simulink model "Encoder_reader_simulink"  (R2025b)
settings: Solver=FixedStepAuto  StartTime=0.0  StopTime=inf  FixedStep=0.0001  RelTol=1e-3  EnableMultiTasking=on
libraries: stm32f4xxblockslib x3, stm32g4xxblockslib x3
settings Model: STM32="{\"EncoderBlockForG4\":[{\"ID\":\"untitled:1\"},{\"ID\":\"Lab3_Encoder:1\"},{\"ID\":\"Encoder_reader_simulink:1\"},{\"ID\":\"Encoder_reader_simulink:58\"},{\"ID\":\"Encoder_reader_simulink:64\"}],\"DigitalPortRead\":[{\"ID\":\"Encoder_reader_simulink:27\"},{\"ID\":\"Encoder_reader_simulink:61\"},{\"ID\":\"Encoder_reader_simulink:62\"}]}"  Creator=User  LastModifiedBy=Asus
settings OptimizationCC: DefaultParameterBehavior=Inlined  EnhancedBackFolding=on  PassReuseOutputArgsAs=Individual arguments  ZeroExternalMemoryAtStartup=off  ZeroInternalMemoryAtStartup=off  MaxStackSize=512  OptimizeBlockOrder=speed  DifferentSizesBufferReuse=on  OptimizationCustomize=off  EfficientTunableParamExpr=on
settings DebuggingCC: ParameterTunabilityLossMsg=error
settings HardwareCC: ProdBitPerPointer=32.0  ProdBitPerSizeT=32.0  ProdBitPerPtrDiffT=32.0  ProdLargestAtomicInteger=Long  ProdLargestAtomicFloat=Double  ProdWordSize=32.0  ProdLongLongMode=on  ProdHWDeviceType=ARM Compatible->ARM Cortex-M
settings SFSimCC: MATLABDynamicMemAlloc=off
settings RTWCC: SystemTargetFile=ert.tlc  HardwareBoard=STM32G4xx Based  TemplateMakefile=ert_default_tmf  Toolchain=GNU Tools for ARM Embedded Processors  Description=Embedded Coder
settings CodeAppCC: ForceParamTrailComments=on  IgnoreCustomStorageClasses=off  OperatorAnnotations=on  SimulinkDataObjDesc=on  SFDataObjDesc=on  InsertBlockDesc=on
settings ERTTargetCC: ExtModeTransport=3.0  ExtModeStaticAlloc=on  ExtModeStaticAllocSize=2048.0  ExtModeMexFile=ext_xcp  ExtModeIntrfLevel=Level2 - Open  TargetLangStandard=C99 (ISO)  CodeReplacementLibrary=ARM Cortex-M  SupportContinuousTime=on

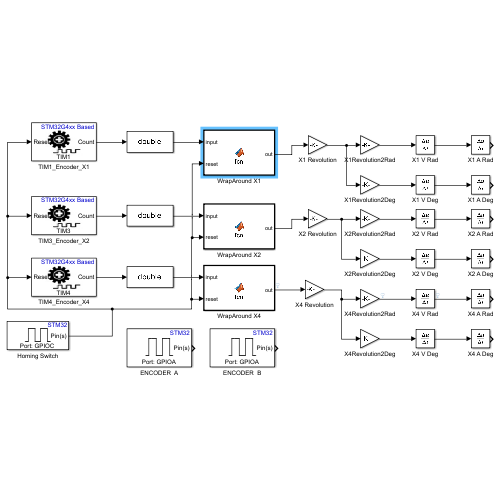
[thumbnail: Simulink's stored preview of the top-level diagram]
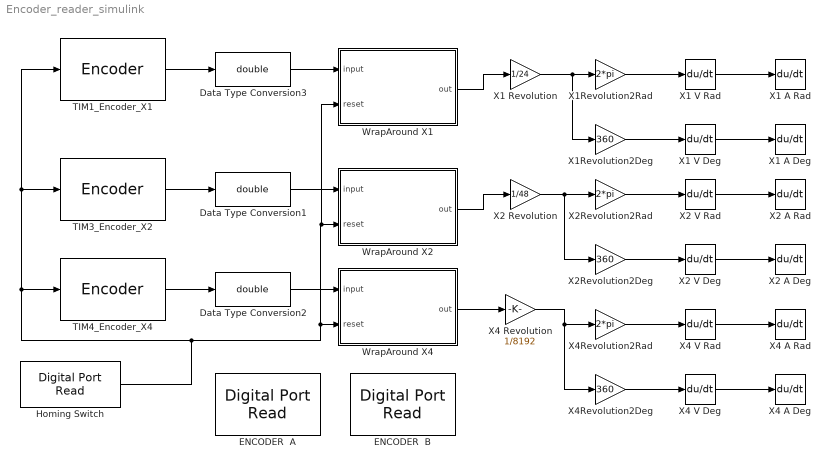
== system Encoder_reader_simulink ==
  Data Type Conversion1 : DataTypeConversion  OutDataTypeStr=double  SaturateOnIntegerOverflow=off  RndMeth=Floor
  Data Type Conversion2 : DataTypeConversion  OutDataTypeStr=double  SaturateOnIntegerOverflow=off  RndMeth=Floor
  Data Type Conversion3 : DataTypeConversion  OutDataTypeStr=double  SaturateOnIntegerOverflow=off  RndMeth=Floor
  ENCODER  A : stm32f4xxblockslib/Digital Port Read  PortName=GPIOA  PinNumber=[6]  ReadOperation=on  IOAsArray=on  SampleTime=-1  EnableSimPort=off  hoistedMaskSrc=ECSoC/ECSimCodegen/Digital Port Read
      settings: LibrarySourceBlock=stm32g4xxblockslib/Digital Port Read
  ENCODER  B : stm32f4xxblockslib/Digital Port Read  PortName=GPIOA  PinNumber=[7]  ReadOperation=on  IOAsArray=on  SampleTime=-1  EnableSimPort=off  hoistedMaskSrc=ECSoC/ECSimCodegen/Digital Port Read
      settings: LibrarySourceBlock=stm32g4xxblockslib/Digital Port Read
  Homing Switch : stm32f4xxblockslib/Digital Port Read  PortName=GPIOC  PinNumber=[13]  ReadOperation=on  IOAsArray=on  SampleTime=-1  EnableSimPort=off  hoistedMaskSrc=ECSoC/ECSimCodegen/Digital Port Read
      settings: LibrarySourceBlock=stm32g4xxblockslib/Digital Port Read
  TIM1_Encoder_X1 : stm32g4xxblockslib/Encoder  TimerModule=TIM1  EnableResetInput=on  OutputCountAfterFirstIndex=off  OutputValidIndex=off  OutputDirection=off  OutputStatus=off  SampleTime=-1
  TIM3_Encoder_X2 : stm32g4xxblockslib/Encoder  TimerModule=TIM3  EnableResetInput=on  OutputCountAfterFirstIndex=off  OutputValidIndex=off  OutputDirection=off  OutputStatus=off  SampleTime=-1
  TIM4_Encoder_X4 : stm32g4xxblockslib/Encoder  TimerModule=TIM4  EnableResetInput=on  OutputCountAfterFirstIndex=off  OutputValidIndex=off  OutputDirection=off  OutputStatus=off  SampleTime=-1
  WrapAround X1 : MATLAB Function  TreatAsAtomicUnit=on
  WrapAround X2 : MATLAB Function  TreatAsAtomicUnit=on
  WrapAround X4 : MATLAB Function  TreatAsAtomicUnit=on
  X1 A Deg : Derivative
  X1 A Rad : Derivative
  X1 Revolution : Gain  Gain=1/24
  X1 V Deg : Derivative
  X1 V Rad : Derivative
  X1Revolution2Deg : Gain  Gain=360
  X1Revolution2Rad : Gain  Gain=2*pi
  X2 A Deg : Derivative
  X2 A Rad : Derivative
  X2 Revolution : Gain  Gain=1/48
  X2 V Deg : Derivative
  X2 V Rad : Derivative
  X2Revolution2Deg : Gain  Gain=360
  X2Revolution2Rad : Gain  Gain=2*pi
  X4 A Deg : Derivative
  X4 A Rad : Derivative
  X4 Revolution : Gain  Gain=1/8192
  X4 V Deg : Derivative
  X4 V Rad : Derivative
  X4Revolution2Deg : Gain  Gain=360
  X4Revolution2Rad : Gain  Gain=2*pi
  wires:
  TIM3_Encoder_X2/1 -> Data Type Conversion1/1
  Data Type Conversion1/1 -> WrapAround X2/1(input)
  X2 V Rad/1 -> X2 A Rad/1
  WrapAround X2/1(out) -> X2 Revolution/1
  X2Revolution2Rad/1 -> X2 V Rad/1
  X2Revolution2Deg/1 -> X2 V Deg/1
  X2 V Deg/1 -> X2 A Deg/1
  Homing Switch/1 -> TIM4_Encoder_X4/1, TIM3_Encoder_X2/1, TIM1_Encoder_X1/1, WrapAround X1/2(reset), WrapAround X2/2(reset), WrapAround X4/2(reset)
  Data Type Conversion2/1 -> WrapAround X4/1(input)
  TIM4_Encoder_X4/1 -> Data Type Conversion2/1
  TIM1_Encoder_X1/1 -> Data Type Conversion3/1
  Data Type Conversion3/1 -> WrapAround X1/1(input)
  X1Revolution2Deg/1 -> X1 V Deg/1
  X1 V Rad/1 -> X1 A Rad/1
  X1 V Deg/1 -> X1 A Deg/1
  X1Revolution2Rad/1 -> X1 V Rad/1
  X4Revolution2Deg/1 -> X4 V Deg/1
  X4 V Rad/1 -> X4 A Rad/1
  X4 V Deg/1 -> X4 A Deg/1
  WrapAround X4/1(out) -> X4 Revolution/1
  X4Revolution2Rad/1 -> X4 V Rad/1
  WrapAround X1/1(out) -> X1 Revolution/1
  X1 Revolution/1 -> X1Revolution2Deg/1, X1Revolution2Rad/1
  X2 Revolution/1 -> X2Revolution2Deg/1, X2Revolution2Rad/1
  X4 Revolution/1 -> X4Revolution2Deg/1, X4Revolution2Rad/1

== matlab function Encoder_reader_simulink/WrapAround X4 ==
  data: input input; out output; reset input
function out = fcn(input, reset)
persistent carry;
persistent preV;
persistent offset;
if isempty(carry)
    carry = 0; 
end 
if isempty(preV)
    preV = 0;
end 
if isempty(offset)
    offset = 0;
end 

diff = input - preV; 
if diff > 30720
    carry = carry - 1;
elseif diff < -30720
    carry = carry + 1;
end 

if reset == 1 
    offset = input + (carry * 61440);
end

preV = input;
out = input + (carry * 61440) - offset;

== matlab function Encoder_reader_simulink/WrapAround X2 ==
  data: input input; out output; reset input
function out = fcn(input, reset)
persistent carry;
persistent preV;
persistent offset;
if isempty(carry)
    carry = 0; 
end 
if isempty(preV)
    preV = 0;
end 
if isempty(offset)
    offset = 0;
end 

diff = input - preV; 
if diff > 30720
    carry = carry - 1;
elseif diff < -30720
    carry = carry + 1;
end 

if reset == 1 
    offset = input + (carry * 61440);
end

preV = input;
out = input + (carry * 61440) - offset;

== matlab function Encoder_reader_simulink/WrapAround X1 ==
  data: input input; out output; reset input
function out = fcn(input, reset)
persistent carry;
persistent preV;
persistent offset;
if isempty(carry)
    carry = 0; 
end 
if isempty(preV)
    preV = 0;
end 
if isempty(offset)
    offset = 0;
end 

diff = input - preV; 
if diff > 30720
    carry = carry - 1;
elseif diff < -30720
    carry = carry + 1;
end 

if reset == 1 
    offset = input + (carry * 61440);
end

preV = input;
out = input + (carry * 61440) - offset;
